simulink model "alternatesim2"  (Simulink 9.3)
settings: Solver=FixedStepAuto  StartTime=0.0  StopTime=9  RelTol=1e-3
libraries: neural x1
settings Model: Creator=Lenovo  LastModifiedBy=Lenovo
settings DataIOCC: SaveFormat=Dataset  SignalLoggingSaveFormat=Dataset  ReturnWorkspaceOutputs=on
settings OptimizationCC: LifeSpan=auto
settings DebuggingCC: UnderspecifiedInitializationDetection=Simplified  MergeDetectMultiDrivingBlocksExec=error  FcnCallInpInsideContextMsg=error  SFUnexpectedBacktrackingDiag=error  SFNoUnconditionalDefaultTransitionDiag=error  SFExecutionAtInitializationDiag=warning  ArithmeticOperatorsInVariantConditions=error
settings HardwareCC: ProdBitPerPointer=64  ProdBitPerSizeT=64  ProdBitPerPtrDiffT=64  ProdLargestAtomicFloat=Float  ProdIntDivRoundTo=Zero  ProdEndianess=LittleEndian  ProdWordSize=64  ProdHWDeviceType=Intel->x86-64 (Windows64)
settings ModelReferenceCC: PropagateSignalLabelsOutOfModel=on
settings SFSimCC: SimUseLocalCustomCode=on
settings RTWCC: RTWUseLocalCustomCode=on
settings CodeAppCC: StateflowObjectComments=off
settings GRTTargetCC: TargetLangStandard=C99 (ISO)  CombineOutputUpdateFcns=on  GRTInterface=off
settings ConfigComp: CovMetricSettings=dwe  CovHtmlReporting=off  CovSaveCumulativeToWorkspaceVar=off  CovSaveSingleToWorkspaceVar=off  CovExternalEMLEnable=on

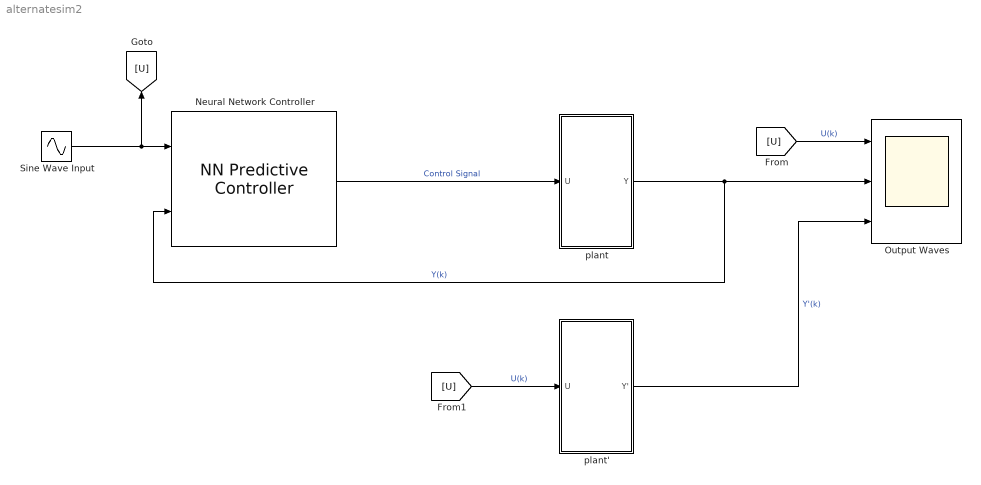
== system alternatesim2 ==
  Neural Network Controller : neural/Control Systems/NN Predictive Controller  epochs=150  minp=-0.99739886259880772279  maxp=0.9951206990243781636  mint=-0.20694236844473831716  maxt=0.9951206990243781636  Normalize=0  IW=[-0.53081199345183216476 -0.18920779506005197534;-1.3649189091330478085 0.14265567100819934176;0.34088554971715850916 -0.61553341859255383817;0.20330495091351691306 -0.94718180487281533608;-1.0593990035718148235 -0.07479909684147045823;0.5532079563247974674 -0.19420903013550769312;0.98302604121762349187 -0.4495985006532601802]  LW1_2=[0.68503510152178914705 -0.033435588029458569725;-0.0015694676008003801033 -0.082920735044702195693;-0.0098341820920744681817 -0.32912503225329747814;-0.25682099374227407296 -0.14149450844160468832;1.1557775942646582035 -0.21395216277716080922;-1.4183639217680186206 0.4445555460125255598;1.6955462798811311576 -0.1972231459520930319]  LW2_1=[1.1447238434060187373 2.7297116831212191457 -0.95319418977111392 0.77892067687991839442 -2.8296864408206703345 -0.93707873890328396982 1.5585784943528213642]  B1=[-1.4393051985938700721;-0.99155916282388067984;0.0028614580403628145366;0.1378900739890584759;-0.79914673694171689533;0.71525063013007739166;0.75281354147453061199]  B2=0.6939997006024308801  max_i_int=15  min_i_int=3  limit_output=0  max_output=Inf  min_output=-Inf  Use_Previous_Weights=1  N2=10  Nu=2  Ts=0.2  rho=0.05  alpha=0.001  csrchfun=csrchbac  maxiter=2  S1=7  Ni=2  Nj=2  sim_file=plant2  trainfun=trainbr  Use_validation=1  Use_Testing=0  max_i=1  min_i=-1  sam_training=10000
      settings: SourceProductName=MATLAB Runtime - Deep Learning Toolbox  SourceProductBaseCode=Missing
  Output Waves : Scope  NumInputPorts=3
  Sine Wave Input : Sin  Amplitude=0.8  Frequency=2  SampleTime=0.2
  plant : Subsystem
  plant' : Subsystem
  wires:
  plant/1("Y ") -> Neural Network Controller/2, Output Waves/2  "Y(k)"
  Neural Network Controller/1 -> plant/1(U)  "Control Signal"
  [U] -> Output Waves/1  "U(k)"
  [U] -> plant'/1(U)  "U(k)"
  plant'/1("Y' ") -> Output Waves/3  "Y'(k)"
  Sine Wave Input/1 -> [U], Neural Network Controller/1

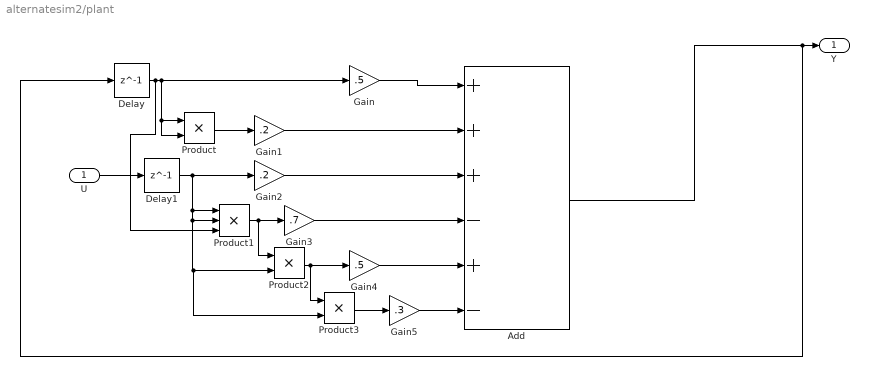
== system alternatesim2/plant ==
  U : Inport
  Add : Sum  Inputs=+++-+-
  Delay : Delay  DelayLength=1  InitialCondition=0
  Delay1 : Delay  DelayLength=1  InitialCondition=0
  Gain : Gain  Gain=.5
  Gain1 : Gain  Gain=.2
  Gain2 : Gain  Gain=.2
  Gain3 : Gain  Gain=.7
  Gain4 : Gain  Gain=.5
  Gain5 : Gain  Gain=.3
  Product : Product
  Product1 : Product  Inputs=3
  Product2 : Product
  Product3 : Product
  "Y " : Outport
  wires:
  Delay/1 -> Product1/3, Product/2, Product/1, Gain/1
  U/1 -> Delay1/1
  Gain5/1 -> Add/6
  Gain2/1 -> Add/3
  Product3/1 -> Gain5/1
  Add/1 -> Delay/1, "Y "/1
  Gain4/1 -> Add/5
  Product2/1 -> Product3/1, Gain4/1
  Delay1/1 -> Product3/2, Product2/2, Product1/2, Product1/1, Gain2/1
  Gain3/1 -> Add/4
  Product1/1 -> Product2/1, Gain3/1
  Gain/1 -> Add/1
  Product/1 -> Gain1/1
  Gain1/1 -> Add/2

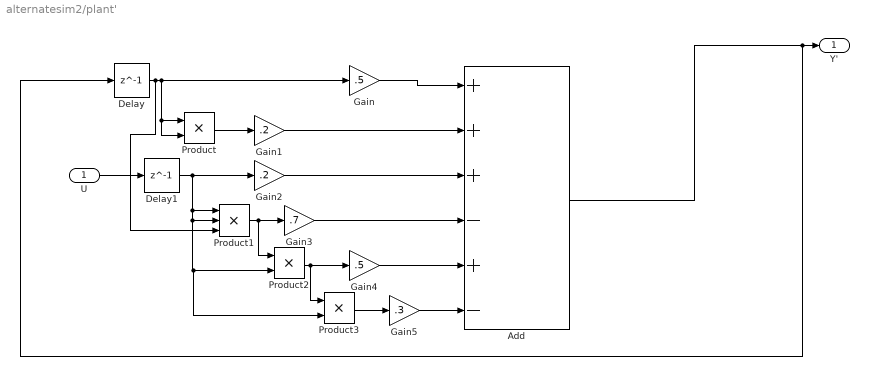
== system alternatesim2/plant' ==
  U : Inport
  Add : Sum  Inputs=+++-+-
  Delay : Delay  DelayLength=1  InitialCondition=0
  Delay1 : Delay  DelayLength=1  InitialCondition=0
  Gain : Gain  Gain=.5
  Gain1 : Gain  Gain=.2
  Gain2 : Gain  Gain=.2
  Gain3 : Gain  Gain=.7
  Gain4 : Gain  Gain=.5
  Gain5 : Gain  Gain=.3
  Product : Product
  Product1 : Product  Inputs=3
  Product2 : Product
  Product3 : Product
  "Y' " : Outport
  wires:
  Delay/1 -> Product1/3, Product/2, Product/1, Gain/1
  U/1 -> Delay1/1
  Gain5/1 -> Add/6
  Gain2/1 -> Add/3
  Product3/1 -> Gain5/1
  Add/1 -> Delay/1, "Y' "/1
  Gain4/1 -> Add/5
  Product2/1 -> Product3/1, Gain4/1
  Delay1/1 -> Product3/2, Product2/2, Product1/2, Product1/1, Gain2/1
  Gain3/1 -> Add/4
  Product1/1 -> Product2/1, Gain3/1
  Gain/1 -> Add/1
  Product/1 -> Gain1/1
  Gain1/1 -> Add/2
